simulink model "Energy_Cost"  (Simulink 8.8)
settings: Solver=ode23t  StartTime=0.0  StopTime=24  RelTol=1e-3  EnableMultiTasking=on
model workspace: external: MAT-File (data not in the file)
libraries: simulink x4
(part 5 of 5)

== system Energy_Cost/Battery/Enabled Subsystem1/Subsystem20 ==
  In1 : Inport
  In2 : Inport  Port=2
  Clock2 : Clock
  Divide26 : Product  Inputs=*/
  Dot Product2 : DotProduct  InputSameDT=on  OutDataTypeStr=Inherit: Inherit via internal rule
  Logical Operator19 : Logic  AllPortsSameDT=off  OutDataTypeStr=boolean
  Relational Operator2 : RelationalOperator  RndMeth=Nearest  InputSameDT=on
  Relational Operator3 : RelationalOperator  Operator=<  RndMeth=Nearest  InputSameDT=on
  Sum : Sum  Inputs=|++
  Sum1 : Sum  Inputs=|-+
  Sum2 : Sum  Inputs=|+-
  Switch2 : Switch  Criteria=u2 > Threshold
  Type1 : Constant  Value=20
  Type54 : Constant
  Type57 : Constant  Value=20
  Type58 : Constant  Value=21
  soc1 : Scope
  Out1 : Outport
  wires:
  Switch2/1 -> Out1/1, soc1/1
  In2/1 -> Sum1/2
  In1/1 -> Sum1/1, Sum/1
  Logical Operator19/1 -> Switch2/2
  Relational Operator3/1 -> Logical Operator19/2
  Type58/1 -> Relational Operator3/2
  Relational Operator2/1 -> Logical Operator19/1
  Type57/1 -> Relational Operator2/2
  Sum/1 -> Switch2/1
  Dot Product2/1 -> Sum/2
  Divide26/1 -> Dot Product2/1
  Type54/1 -> Divide26/2
  Sum1/1 -> Divide26/1
  Clock2/1 -> Sum2/1, Relational Operator2/1, Relational Operator3/1
  Type1/1 -> Sum2/2
  Sum2/1 -> Dot Product2/2

== system Energy_Cost/Battery/Enabled Subsystem1/Subsystem21 ==
  In1 : Inport
  In2 : Inport  Port=2
  Clock2 : Clock
  Divide26 : Product  Inputs=*/
  Dot Product2 : DotProduct  InputSameDT=on  OutDataTypeStr=Inherit: Inherit via internal rule
  Logical Operator19 : Logic  AllPortsSameDT=off  OutDataTypeStr=boolean
  Relational Operator2 : RelationalOperator  RndMeth=Nearest  InputSameDT=on
  Relational Operator3 : RelationalOperator  Operator=<  RndMeth=Nearest  InputSameDT=on
  Sum : Sum  Inputs=|++
  Sum1 : Sum  Inputs=|-+
  Sum2 : Sum  Inputs=|+-
  Switch2 : Switch  Criteria=u2 > Threshold
  Type1 : Constant  Value=21
  Type54 : Constant
  Type57 : Constant  Value=21
  Type58 : Constant  Value=22
  soc1 : Scope
  Out1 : Outport
  wires:
  Sum2/1 -> Dot Product2/2
  Type1/1 -> Sum2/2
  Clock2/1 -> Relational Operator3/1, Relational Operator2/1, Sum2/1
  Sum1/1 -> Divide26/1
  Type54/1 -> Divide26/2
  Divide26/1 -> Dot Product2/1
  Dot Product2/1 -> Sum/2
  Sum/1 -> Switch2/1
  Type57/1 -> Relational Operator2/2
  Relational Operator2/1 -> Logical Operator19/1
  Type58/1 -> Relational Operator3/2
  Relational Operator3/1 -> Logical Operator19/2
  Logical Operator19/1 -> Switch2/2
  In1/1 -> Sum/1, Sum1/1
  In2/1 -> Sum1/2
  Switch2/1 -> soc1/1, Out1/1

== system Energy_Cost/Battery/Enabled Subsystem1/Subsystem22 ==
  In1 : Inport
  In2 : Inport  Port=2
  Clock2 : Clock
  Divide26 : Product  Inputs=*/
  Dot Product2 : DotProduct  InputSameDT=on  OutDataTypeStr=Inherit: Inherit via internal rule
  Logical Operator19 : Logic  AllPortsSameDT=off  OutDataTypeStr=boolean
  Relational Operator2 : RelationalOperator  RndMeth=Nearest  InputSameDT=on
  Relational Operator3 : RelationalOperator  Operator=<  RndMeth=Nearest  InputSameDT=on
  Sum : Sum  Inputs=|++
  Sum1 : Sum  Inputs=|-+
  Sum2 : Sum  Inputs=|+-
  Switch2 : Switch  Criteria=u2 > Threshold
  Type1 : Constant  Value=22
  Type54 : Constant
  Type57 : Constant  Value=22
  Type58 : Constant  Value=23
  soc1 : Scope
  Out1 : Outport
  wires:
  Switch2/1 -> Out1/1, soc1/1
  In2/1 -> Sum1/2
  In1/1 -> Sum1/1, Sum/1
  Logical Operator19/1 -> Switch2/2
  Relational Operator3/1 -> Logical Operator19/2
  Type58/1 -> Relational Operator3/2
  Relational Operator2/1 -> Logical Operator19/1
  Type57/1 -> Relational Operator2/2
  Sum/1 -> Switch2/1
  Dot Product2/1 -> Sum/2
  Divide26/1 -> Dot Product2/1
  Type54/1 -> Divide26/2
  Sum1/1 -> Divide26/1
  Clock2/1 -> Sum2/1, Relational Operator2/1, Relational Operator3/1
  Type1/1 -> Sum2/2
  Sum2/1 -> Dot Product2/2

== system Energy_Cost/Battery/Enabled Subsystem1/Subsystem23 ==
  In1 : Inport
  In2 : Inport  Port=2
  Clock2 : Clock
  Divide26 : Product  Inputs=*/
  Dot Product2 : DotProduct  InputSameDT=on  OutDataTypeStr=Inherit: Inherit via internal rule
  Logical Operator19 : Logic  AllPortsSameDT=off  OutDataTypeStr=boolean
  Relational Operator2 : RelationalOperator  RndMeth=Nearest  InputSameDT=on
  Relational Operator3 : RelationalOperator  Operator=<  RndMeth=Nearest  InputSameDT=on
  Sum : Sum  Inputs=|++
  Sum1 : Sum  Inputs=|-+
  Sum2 : Sum  Inputs=|+-
  Switch2 : Switch  Criteria=u2 > Threshold
  Type1 : Constant  Value=23
  Type54 : Constant
  Type57 : Constant  Value=23
  Type58 : Constant  Value=24
  soc1 : Scope
  Out1 : Outport
  wires:
  Sum2/1 -> Dot Product2/2
  Type1/1 -> Sum2/2
  Clock2/1 -> Relational Operator3/1, Relational Operator2/1, Sum2/1
  Sum1/1 -> Divide26/1
  Type54/1 -> Divide26/2
  Divide26/1 -> Dot Product2/1
  Dot Product2/1 -> Sum/2
  Sum/1 -> Switch2/1
  Type57/1 -> Relational Operator2/2
  Relational Operator2/1 -> Logical Operator19/1
  Type58/1 -> Relational Operator3/2
  Relational Operator3/1 -> Logical Operator19/2
  Logical Operator19/1 -> Switch2/2
  In1/1 -> Sum/1, Sum1/1
  In2/1 -> Sum1/2
  Switch2/1 -> soc1/1, Out1/1

== system Energy_Cost/Battery/Enabled Subsystem1/Subsystem3 ==
  In1 : Inport
  In2 : Inport  Port=2
  Clock2 : Clock
  Divide26 : Product  Inputs=*/
  Dot Product2 : DotProduct  InputSameDT=on  OutDataTypeStr=Inherit: Inherit via internal rule
  Logical Operator19 : Logic  AllPortsSameDT=off  OutDataTypeStr=boolean
  Relational Operator2 : RelationalOperator  RndMeth=Nearest  InputSameDT=on
  Relational Operator3 : RelationalOperator  Operator=<  RndMeth=Nearest  InputSameDT=on
  Sum : Sum  Inputs=|++
  Sum1 : Sum  Inputs=|-+
  Sum2 : Sum  Inputs=|+-
  Switch2 : Switch  Criteria=u2 > Threshold
  Type1 : Constant  Value=3
  Type54 : Constant
  Type57 : Constant  Value=3
  Type58 : Constant  Value=4
  soc1 : Scope
  Out1 : Outport
  wires:
  Switch2/1 -> Out1/1, soc1/1
  In2/1 -> Sum1/2
  In1/1 -> Sum1/1, Sum/1
  Logical Operator19/1 -> Switch2/2
  Relational Operator3/1 -> Logical Operator19/2
  Type58/1 -> Relational Operator3/2
  Relational Operator2/1 -> Logical Operator19/1
  Type57/1 -> Relational Operator2/2
  Sum/1 -> Switch2/1
  Dot Product2/1 -> Sum/2
  Divide26/1 -> Dot Product2/1
  Type54/1 -> Divide26/2
  Sum1/1 -> Divide26/1
  Clock2/1 -> Sum2/1, Relational Operator2/1, Relational Operator3/1
  Type1/1 -> Sum2/2
  Sum2/1 -> Dot Product2/2

== system Energy_Cost/Battery/Enabled Subsystem1/Subsystem4 ==
  In1 : Inport
  In2 : Inport  Port=2
  Clock2 : Clock
  Divide26 : Product  Inputs=*/
  Dot Product2 : DotProduct  InputSameDT=on  OutDataTypeStr=Inherit: Inherit via internal rule
  Logical Operator19 : Logic  AllPortsSameDT=off  OutDataTypeStr=boolean
  Relational Operator2 : RelationalOperator  RndMeth=Nearest  InputSameDT=on
  Relational Operator3 : RelationalOperator  Operator=<  RndMeth=Nearest  InputSameDT=on
  Sum : Sum  Inputs=|++
  Sum1 : Sum  Inputs=|-+
  Sum2 : Sum  Inputs=|+-
  Switch2 : Switch  Criteria=u2 > Threshold
  Type1 : Constant  Value=4
  Type54 : Constant
  Type57 : Constant  Value=4
  Type58 : Constant  Value=5
  soc1 : Scope
  Out1 : Outport
  wires:
  Sum2/1 -> Dot Product2/2
  Type1/1 -> Sum2/2
  Clock2/1 -> Relational Operator3/1, Relational Operator2/1, Sum2/1
  Sum1/1 -> Divide26/1
  Type54/1 -> Divide26/2
  Divide26/1 -> Dot Product2/1
  Dot Product2/1 -> Sum/2
  Sum/1 -> Switch2/1
  Type57/1 -> Relational Operator2/2
  Relational Operator2/1 -> Logical Operator19/1
  Type58/1 -> Relational Operator3/2
  Relational Operator3/1 -> Logical Operator19/2
  Logical Operator19/1 -> Switch2/2
  In1/1 -> Sum/1, Sum1/1
  In2/1 -> Sum1/2
  Switch2/1 -> soc1/1, Out1/1

== system Energy_Cost/Battery/Enabled Subsystem1/Subsystem5 ==
  In1 : Inport
  In2 : Inport  Port=2
  Clock2 : Clock
  Divide26 : Product  Inputs=*/
  Dot Product2 : DotProduct  InputSameDT=on  OutDataTypeStr=Inherit: Inherit via internal rule
  Logical Operator19 : Logic  AllPortsSameDT=off  OutDataTypeStr=boolean
  Relational Operator2 : RelationalOperator  RndMeth=Nearest  InputSameDT=on
  Relational Operator3 : RelationalOperator  Operator=<  RndMeth=Nearest  InputSameDT=on
  Sum : Sum  Inputs=|++
  Sum1 : Sum  Inputs=|-+
  Sum2 : Sum  Inputs=|+-
  Switch2 : Switch  Criteria=u2 > Threshold
  Type1 : Constant  Value=5
  Type54 : Constant
  Type57 : Constant  Value=5
  Type58 : Constant  Value=6
  soc1 : Scope
  Out1 : Outport
  wires:
  Switch2/1 -> Out1/1, soc1/1
  In2/1 -> Sum1/2
  In1/1 -> Sum1/1, Sum/1
  Logical Operator19/1 -> Switch2/2
  Relational Operator3/1 -> Logical Operator19/2
  Type58/1 -> Relational Operator3/2
  Relational Operator2/1 -> Logical Operator19/1
  Type57/1 -> Relational Operator2/2
  Sum/1 -> Switch2/1
  Dot Product2/1 -> Sum/2
  Divide26/1 -> Dot Product2/1
  Type54/1 -> Divide26/2
  Sum1/1 -> Divide26/1
  Clock2/1 -> Sum2/1, Relational Operator2/1, Relational Operator3/1
  Type1/1 -> Sum2/2
  Sum2/1 -> Dot Product2/2

== system Energy_Cost/Battery/Enabled Subsystem1/Subsystem6 ==
  In1 : Inport
  In2 : Inport  Port=2
  Clock2 : Clock
  Divide26 : Product  Inputs=*/
  Dot Product2 : DotProduct  InputSameDT=on  OutDataTypeStr=Inherit: Inherit via internal rule
  Logical Operator19 : Logic  AllPortsSameDT=off  OutDataTypeStr=boolean
  Relational Operator2 : RelationalOperator  RndMeth=Nearest  InputSameDT=on
  Relational Operator3 : RelationalOperator  Operator=<  RndMeth=Nearest  InputSameDT=on
  Sum : Sum  Inputs=|++
  Sum1 : Sum  Inputs=|-+
  Sum2 : Sum  Inputs=|+-
  Switch2 : Switch  Criteria=u2 > Threshold
  Type1 : Constant  Value=6
  Type54 : Constant
  Type57 : Constant  Value=6
  Type58 : Constant  Value=7
  soc1 : Scope
  Out1 : Outport
  wires:
  Sum2/1 -> Dot Product2/2
  Type1/1 -> Sum2/2
  Clock2/1 -> Relational Operator3/1, Relational Operator2/1, Sum2/1
  Sum1/1 -> Divide26/1
  Type54/1 -> Divide26/2
  Divide26/1 -> Dot Product2/1
  Dot Product2/1 -> Sum/2
  Sum/1 -> Switch2/1
  Type57/1 -> Relational Operator2/2
  Relational Operator2/1 -> Logical Operator19/1
  Type58/1 -> Relational Operator3/2
  Relational Operator3/1 -> Logical Operator19/2
  Logical Operator19/1 -> Switch2/2
  In1/1 -> Sum/1, Sum1/1
  In2/1 -> Sum1/2
  Switch2/1 -> soc1/1, Out1/1

== system Energy_Cost/Battery/Enabled Subsystem1/Subsystem7 ==
  In1 : Inport
  In2 : Inport  Port=2
  Clock2 : Clock
  Divide26 : Product  Inputs=*/
  Dot Product2 : DotProduct  InputSameDT=on  OutDataTypeStr=Inherit: Inherit via internal rule
  Logical Operator19 : Logic  AllPortsSameDT=off  OutDataTypeStr=boolean
  Relational Operator2 : RelationalOperator  RndMeth=Nearest  InputSameDT=on
  Relational Operator3 : RelationalOperator  Operator=<  RndMeth=Nearest  InputSameDT=on
  Sum : Sum  Inputs=|++
  Sum1 : Sum  Inputs=|-+
  Sum2 : Sum  Inputs=|+-
  Switch2 : Switch  Criteria=u2 > Threshold
  Type1 : Constant  Value=7
  Type54 : Constant
  Type57 : Constant  Value=7
  Type58 : Constant  Value=8
  soc1 : Scope
  Out1 : Outport
  wires:
  Switch2/1 -> Out1/1, soc1/1
  In2/1 -> Sum1/2
  In1/1 -> Sum1/1, Sum/1
  Logical Operator19/1 -> Switch2/2
  Relational Operator3/1 -> Logical Operator19/2
  Type58/1 -> Relational Operator3/2
  Relational Operator2/1 -> Logical Operator19/1
  Type57/1 -> Relational Operator2/2
  Sum/1 -> Switch2/1
  Dot Product2/1 -> Sum/2
  Divide26/1 -> Dot Product2/1
  Type54/1 -> Divide26/2
  Sum1/1 -> Divide26/1
  Clock2/1 -> Sum2/1, Relational Operator2/1, Relational Operator3/1
  Type1/1 -> Sum2/2
  Sum2/1 -> Dot Product2/2

== system Energy_Cost/Battery/Enabled Subsystem1/Subsystem8 ==
  In1 : Inport
  In2 : Inport  Port=2
  Clock2 : Clock
  Divide26 : Product  Inputs=*/
  Dot Product2 : DotProduct  InputSameDT=on  OutDataTypeStr=Inherit: Inherit via internal rule
  Logical Operator19 : Logic  AllPortsSameDT=off  OutDataTypeStr=boolean
  Relational Operator2 : RelationalOperator  RndMeth=Nearest  InputSameDT=on
  Relational Operator3 : RelationalOperator  Operator=<  RndMeth=Nearest  InputSameDT=on
  Sum : Sum  Inputs=|++
  Sum1 : Sum  Inputs=|-+
  Sum2 : Sum  Inputs=|+-
  Switch2 : Switch  Criteria=u2 > Threshold
  Type1 : Constant  Value=8
  Type54 : Constant
  Type57 : Constant  Value=8
  Type58 : Constant  Value=9
  soc1 : Scope
  Out1 : Outport
  wires:
  Sum2/1 -> Dot Product2/2
  Type1/1 -> Sum2/2
  Clock2/1 -> Relational Operator3/1, Relational Operator2/1, Sum2/1
  Sum1/1 -> Divide26/1
  Type54/1 -> Divide26/2
  Divide26/1 -> Dot Product2/1
  Dot Product2/1 -> Sum/2
  Sum/1 -> Switch2/1
  Type57/1 -> Relational Operator2/2
  Relational Operator2/1 -> Logical Operator19/1
  Type58/1 -> Relational Operator3/2
  Relational Operator3/1 -> Logical Operator19/2
  Logical Operator19/1 -> Switch2/2
  In1/1 -> Sum/1, Sum1/1
  In2/1 -> Sum1/2
  Switch2/1 -> soc1/1, Out1/1

== system Energy_Cost/Battery/Enabled Subsystem1/Subsystem9 ==
  In1 : Inport
  In2 : Inport  Port=2
  Clock2 : Clock
  Divide26 : Product  Inputs=*/
  Dot Product2 : DotProduct  InputSameDT=on  OutDataTypeStr=Inherit: Inherit via internal rule
  Logical Operator19 : Logic  AllPortsSameDT=off  OutDataTypeStr=boolean
  Relational Operator2 : RelationalOperator  RndMeth=Nearest  InputSameDT=on
  Relational Operator3 : RelationalOperator  Operator=<  RndMeth=Nearest  InputSameDT=on
  Sum : Sum  Inputs=|++
  Sum1 : Sum  Inputs=|-+
  Sum2 : Sum  Inputs=|+-
  Switch2 : Switch  Criteria=u2 > Threshold
  Type1 : Constant  Value=9
  Type54 : Constant
  Type57 : Constant  Value=9
  Type58 : Constant  Value=10
  soc1 : Scope
  Out1 : Outport
  wires:
  Switch2/1 -> Out1/1, soc1/1
  In2/1 -> Sum1/2
  In1/1 -> Sum1/1, Sum/1
  Logical Operator19/1 -> Switch2/2
  Relational Operator3/1 -> Logical Operator19/2
  Type58/1 -> Relational Operator3/2
  Relational Operator2/1 -> Logical Operator19/1
  Type57/1 -> Relational Operator2/2
  Sum/1 -> Switch2/1
  Dot Product2/1 -> Sum/2
  Divide26/1 -> Dot Product2/1
  Type54/1 -> Divide26/2
  Sum1/1 -> Divide26/1
  Clock2/1 -> Sum2/1, Relational Operator2/1, Relational Operator3/1
  Type1/1 -> Sum2/2
  Sum2/1 -> Dot Product2/2

== system Energy_Cost/House/Room_1/Iinst ==
  Constant : Constant  Value=20
  Constant1 : Constant  Value=5
  Constant2 : Constant  Value=-1
  Constant3 : Constant  Value=600
  Constant4 : Constant  Value=200
  Digital Clock : DigitalClock
  Divide : Product  Inputs=*/
  Heater Switch1 : Product  RndMeth=Zero
  Heater Switch2 : Product  RndMeth=Zero
  Heater Switch3 : Product  RndMeth=Zero
  Math Function1 : Math  SaturateOnIntegerOverflow=on
  Solar : Scope
  Subtract1 : Sum
  Subtract2 : Sum  Inputs=+-
  Iinst : Outport  InitialOutput=0
  wires:
  Digital Clock/1 -> Subtract2/1
  Constant/1 -> Subtract2/2
  Subtract2/1 -> Heater Switch1/1, Heater Switch1/2
  Heater Switch1/1 -> Divide/1
  Constant1/1 -> Divide/2
  Divide/1 -> Heater Switch2/2
  Constant2/1 -> Heater Switch2/1
  Heater Switch2/1 -> Math Function1/1
  Math Function1/1 -> Heater Switch3/2
  Constant3/1 -> Heater Switch3/1
  Subtract1/1 -> Iinst/1, Solar/1
  Constant4/1 -> Subtract1/1
  Heater Switch3/1 -> Subtract1/2

== system Energy_Cost/House/Room_2/Iinst ==
  Clock : Clock
  Constant : Constant  Value=20
  Constant1 : Constant  Value=5
  Constant2 : Constant  Value=-1
  Constant3 : Constant  Value=600
  Constant4 : Constant  Value=200
  Divide : Product  Inputs=*/
  Heater Switch1 : Product  RndMeth=Zero
  Heater Switch2 : Product  RndMeth=Zero
  Heater Switch3 : Product  RndMeth=Zero
  Math Function1 : Math  SaturateOnIntegerOverflow=on
  Solar : Scope
  Subtract1 : Sum
  Subtract2 : Sum  Inputs=+-
  Iinst : Outport  InitialOutput=0
  wires:
  Clock/1 -> Subtract2/1
  Constant/1 -> Subtract2/2
  Subtract2/1 -> Heater Switch1/1, Heater Switch1/2
  Heater Switch1/1 -> Divide/1
  Constant1/1 -> Divide/2
  Divide/1 -> Heater Switch2/2
  Constant2/1 -> Heater Switch2/1
  Heater Switch2/1 -> Math Function1/1
  Math Function1/1 -> Heater Switch3/2
  Constant3/1 -> Heater Switch3/1
  Subtract1/1 -> Iinst/1, Solar/1
  Constant4/1 -> Subtract1/1
  Heater Switch3/1 -> Subtract1/2

== system Energy_Cost/House/Room_3/Iinst ==
  Clock : Clock
  Constant : Constant  Value=20
  Constant1 : Constant  Value=5
  Constant2 : Constant  Value=-1
  Constant3 : Constant  Value=600
  Constant4 : Constant  Value=200
  Divide : Product  Inputs=*/
  Heater Switch1 : Product  RndMeth=Zero
  Heater Switch2 : Product  RndMeth=Zero
  Heater Switch3 : Product  RndMeth=Zero
  Math Function1 : Math  SaturateOnIntegerOverflow=on
  Solar : Scope
  Subtract1 : Sum
  Subtract2 : Sum  Inputs=+-
  Iinst : Outport  InitialOutput=0
  wires:
  Clock/1 -> Subtract2/1
  Constant/1 -> Subtract2/2
  Subtract2/1 -> Heater Switch1/1, Heater Switch1/2
  Heater Switch1/1 -> Divide/1
  Constant1/1 -> Divide/2
  Divide/1 -> Heater Switch2/2
  Constant2/1 -> Heater Switch2/1
  Heater Switch2/1 -> Math Function1/1
  Math Function1/1 -> Heater Switch3/2
  Constant3/1 -> Heater Switch3/1
  Subtract1/1 -> Iinst/1, Solar/1
  Constant4/1 -> Subtract1/1
  Heater Switch3/1 -> Subtract1/2

== system Energy_Cost/House/Room_4/Iinst ==
  Clock : Clock
  Constant : Constant  Value=20
  Constant1 : Constant  Value=5
  Constant2 : Constant  Value=-1
  Constant3 : Constant  Value=600
  Constant4 : Constant  Value=200
  Divide : Product  Inputs=*/
  Heater Switch1 : Product  RndMeth=Zero
  Heater Switch2 : Product  RndMeth=Zero
  Heater Switch3 : Product  RndMeth=Zero
  Math Function1 : Math  SaturateOnIntegerOverflow=on
  Solar : Scope
  Subtract1 : Sum
  Subtract2 : Sum  Inputs=+-
  Iinst : Outport  InitialOutput=0
  wires:
  Clock/1 -> Subtract2/1
  Constant/1 -> Subtract2/2
  Subtract2/1 -> Heater Switch1/1, Heater Switch1/2
  Heater Switch1/1 -> Divide/1
  Constant1/1 -> Divide/2
  Divide/1 -> Heater Switch2/2
  Constant2/1 -> Heater Switch2/1
  Heater Switch2/1 -> Math Function1/1
  Math Function1/1 -> Heater Switch3/2
  Constant3/1 -> Heater Switch3/1
  Subtract1/1 -> Iinst/1, Solar/1
  Constant4/1 -> Subtract1/1
  Heater Switch3/1 -> Subtract1/2
